simulink model "ModelTest"  (R2023b)
settings: Solver=FixedStepDiscrete  StartTime=0.0  StopTime=1  FixedStep=5e-5  RelTol=1e-3  EnableMultiTasking=on
libraries: simulink x1
settings Model: Creator=YXuan  LastModifiedBy=YXuan
settings SolverCC: PositivePriorityOrder=on
settings OptimizationCC: DefaultUnderspecifiedDataType=single

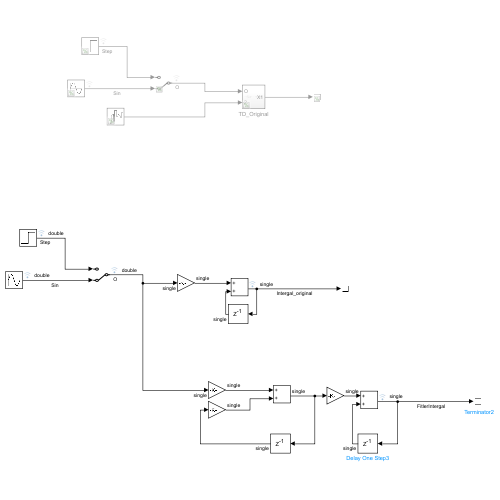
[thumbnail: Simulink's stored preview of the top-level diagram]
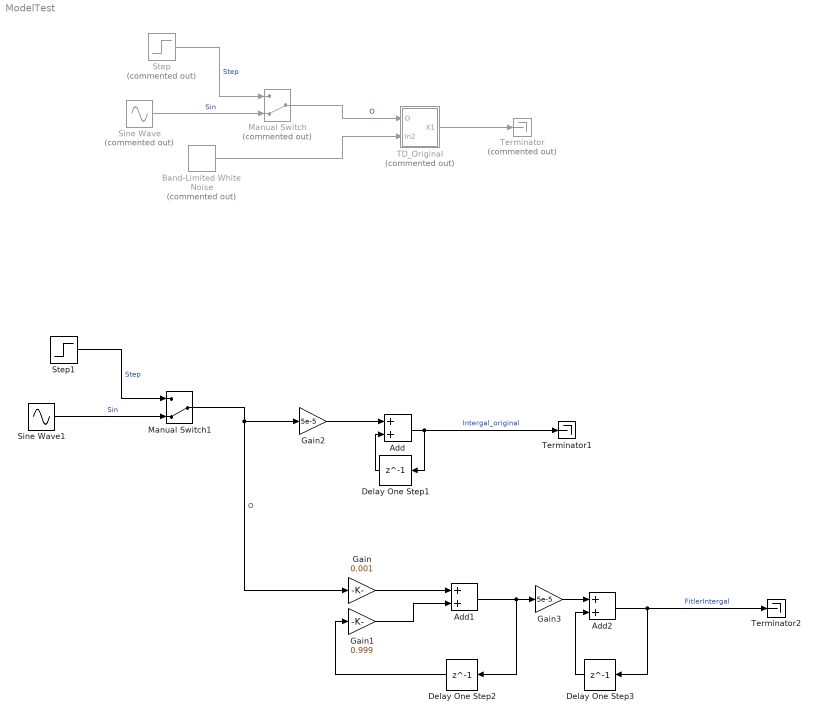
== system ModelTest ==
  Add : Sum
  Add1 : Sum
  Add2 : Sum
  Band-Limited White Noise : simulink/Sources/Band-Limited White Noise  Commented=on  Cov=[0]  Ts=5e-5  seed=[23341]
  Delay One Step1 : Delay  DelayLength=1  InitialCondition=single(0)
  Delay One Step2 : Delay  DelayLength=1  InitialCondition=single(0)
  Delay One Step3 : Delay  DelayLength=1  InitialCondition=single(0)
  Gain : Gain  Gain=0.001
  Gain1 : Gain  Gain=0.999
  Gain2 : Gain  Gain=5e-5
  Gain3 : Gain  Gain=5e-5
  Manual Switch : ManualSwitch  Commented=on  CurrentSetting=0
  Manual Switch1 : ManualSwitch  CurrentSetting=0
  Sine Wave : Sin  Commented=on  Frequency=2*pi*1
  Sine Wave1 : Sin  Frequency=2*pi*1
  Step : Step  Commented=on  OutDataTypeStr=single
  Step1 : Step  OutDataTypeStr=single
  TD_Original : Subsystem  Commented=on
  Terminator : Terminator  Commented=on
  Terminator1 : Terminator
  Terminator2 : Terminator
  wires:
  Step/1 -> Manual Switch/1  "Step"
  Sine Wave/1 -> Manual Switch/2  "Sin"
  Manual Switch/1 -> TD_Original/1(O)  "O"
  Band-Limited White Noise/1 -> TD_Original/2(In2)
  TD_Original/1(X1) -> Terminator/1
  Add/1 -> Terminator1/1, Delay One Step1/1  "Intergal_original"
  Delay One Step1/1 -> Add/2
  Gain/1 -> Add1/1
  Gain1/1 -> Add1/2
  Delay One Step2/1 -> Gain1/1
  Add1/1 -> Gain3/1, Delay One Step2/1
  Gain2/1 -> Add/1
  Add2/1 -> Delay One Step3/1, Terminator2/1  "FitlerIntergal"
  Delay One Step3/1 -> Add2/2
  Gain3/1 -> Add2/1
  Manual Switch1/1 -> Gain/1, Gain2/1  "O"
  Sine Wave1/1 -> Manual Switch1/2  "Sin"
  Step1/1 -> Manual Switch1/1  "Step"

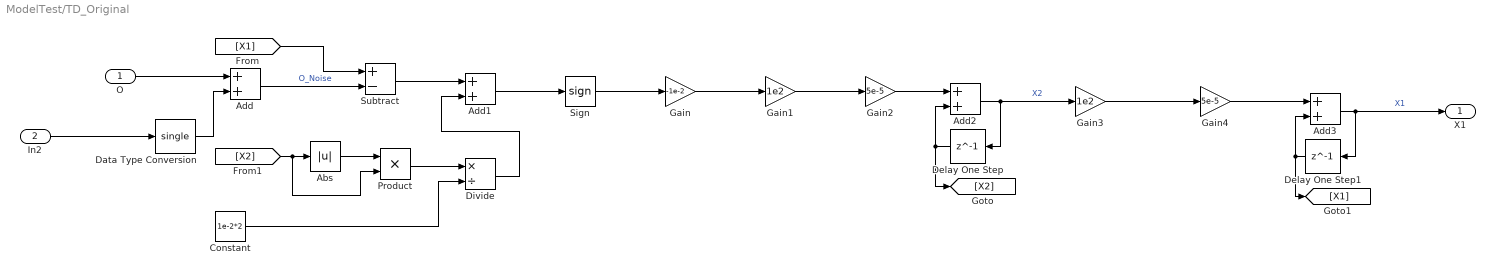
== system ModelTest/TD_Original ==
  O : Inport
  In2 : Inport  Port=2
  Abs : Abs  SaturateOnIntegerOverflow=off
  Add{,1..3} (4 alike) : Sum
  Constant : Constant  Value=1e-2*2
  Data Type Conversion : DataTypeConversion  OutDataTypeStr=single  RndMeth=Simplest  SaturateOnIntegerOverflow=off
  Delay One Step : Delay  DelayLength=1  InitialCondition=single(0)
  Delay One Step1 : Delay  DelayLength=1  InitialCondition=single(0)
  Divide : Product  Inputs=*/
  Gain : Gain  Gain=-1e-2
  Gain1 : Gain  Gain=1e2
  Gain2 : Gain  Gain=5e-5
  Gain3 : Gain  Gain=1e2
  Gain4 : Gain  Gain=5e-5
  Product : Product
  Sign : Signum
  Subtract : Sum  Inputs=+-
  X1 : Outport
  wires:
  Gain3/1 -> Gain4/1
  [X1] -> Subtract/1
  Sign/1 -> Gain/1
  Product/1 -> Divide/1
  Gain1/1 -> Gain2/1
  Add2/1 -> Gain3/1, Delay One Step/1  "X2"
  In2/1 -> Data Type Conversion/1
  Add1/1 -> Sign/1
  Delay One Step1/1 -> Add3/2, [X1]
  Subtract/1 -> Add1/1
  Add/1 -> Subtract/2  "O_Noise"
  O/1 -> Add/1
  Delay One Step/1 -> [X2], Add2/2
  Abs/1 -> Product/1
  Constant/1 -> Divide/2
  Add3/1 -> X1/1, Delay One Step1/1  "X1"
  [X2] -> Product/2, Abs/1
  Gain2/1 -> Add2/1
  Data Type Conversion/1 -> Add/2
  Gain4/1 -> Add3/1
  Divide/1 -> Add1/2
  Gain/1 -> Gain1/1
